simulink model "PID_controller"  (R2023b)
settings: Solver=FixedStepAuto  StartTime=0.0  StopTime=20  FixedStep=0.005  RelTol=1e-3
settings Model: Creator=suvo  LastModifiedBy=suvo
settings SolverCC: AlgebraicLoopSolver=TrustRegion
settings DebuggingCC: UnconnectedInputMsg=warning  UnconnectedOutputMsg=warning  UnconnectedLineMsg=warning
settings ModelReferenceCC: EnableRefExpFcnMdlSchedulingChecks=on

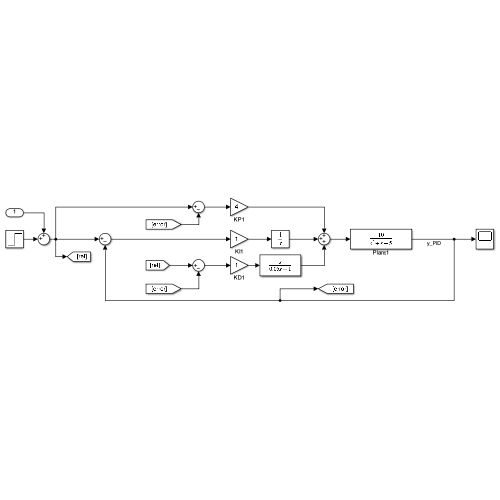
[thumbnail: Simulink's stored preview of the top-level diagram]
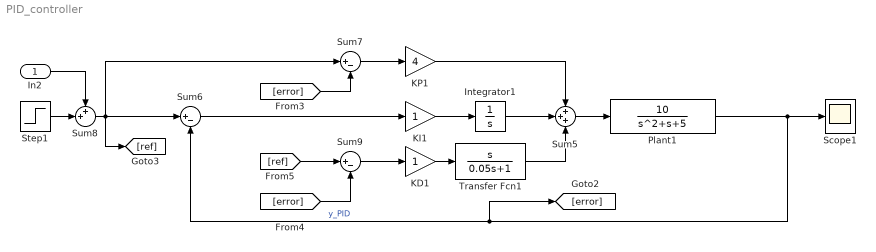
== system PID_controller ==
  In2 : Inport
  Integrator1 : Integrator
  KD1 : Gain
  KI1 : Gain
  KP1 : Gain  Gain=4
  Plant1 : TransferFcn  Numerator=10  Denominator=[1 1 5]
  Scope1 : Scope
  Step1 : Step  SampleTime=0
  Sum5 : Sum  Inputs=+++
  Sum6 : Sum  Inputs=|+-
  Sum7 : Sum  Inputs=|+-
  Sum8 : Sum  Inputs=++|
  Sum9 : Sum  Inputs=|+-
  Transfer Fcn1 : TransferFcn  Numerator=[1 0]  Denominator=[0.05 1]
  wires:
  Transfer Fcn1/1 -> Sum5/3
  [error] -> Sum7/2
  KP1/1 -> Sum5/1
  Integrator1/1 -> Sum5/2
  Sum9/1 -> KD1/1
  Sum8/1 -> Sum7/1, Sum6/1, [ref]
  Sum7/1 -> KP1/1
  In2/1 -> Sum8/1
  Step1/1 -> Sum8/2
  KI1/1 -> Integrator1/1
  Sum5/1 -> Plant1/1
  Sum6/1 -> KI1/1
  KD1/1 -> Transfer Fcn1/1
  Plant1/1 -> Scope1/1, Sum6/2, [error]  "y_PID"
  [error] -> Sum9/2
  [ref] -> Sum9/1
